simulink model "ejh42"  (Simulink 3.00)
settings: Solver=ode45  StartTime=0.0  StopTime=10.0  RelTol=1e-3
settings Model: LastModifiedBy=Administrador

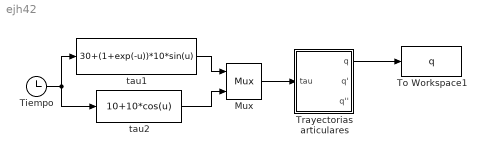
== system ejh42 ==
  Mux : Mux  Inputs=2
      settings: DisplayOption=none
  Tiempo : Clock
      settings: DisplayTime=off  Decimation=10
  To Workspace1 : ToWorkspace  VariableName=q  SampleTime=-1  SaveFormat=Matrix
  Trayectorias articulares : Subsystem  mask(Trayectorias articulares){dyn=[0 0 0 0 0 2 3 0 0 0 0 0 0 0 0 0 1 0 0 0; 0 3 0 0 0 1 1 0 0 0 0 0 0 0 0 0 1 0 0 0], grav=[0 -9.81 0], inivel=[0 0], inipos=[0 0]}
      mask prompts: dyn "Matriz de parámetros cinemáticos y dinámicos:"; grav "Vector aceleración de la gravedad:"; inivel "Velocidades articulares iniciales:"; inipos "Posiciones articulares iniciales:"
      mask help: Se calculan las trayectorias articulares (posiciones, velocidades y aceleraciones articulares) a partir de los pares aplicados al manipulador.
  tau1 : Fcn  Expr=30+(1+exp(-u))*10*sin(u)
  tau2 : Fcn  Expr=10+10*cos(u)
  wires:
  Mux/1 -> Trayectorias articulares/1(tau)
  Trayectorias articulares/1(q) -> To Workspace1/1
  Tiempo/1 -> tau1/1, tau2/1
  tau1/1 -> Mux/1
  tau2/1 -> Mux/2

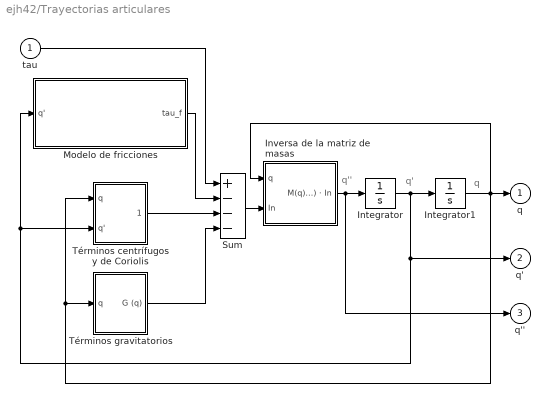
== system ejh42/Trayectorias articulares ==
  note: q
  note: q''
  note: q'
  tau : Inport  Port=1  PortWidth=-1  SampleTime=-1  DataType=auto
      settings: SignalType=auto
  Integrator : Integrator  ExternalReset=none  InitialConditionSource=internal  InitialCondition=inivel(:)  LimitOutput=off  UpperSaturationLimit=inf  LowerSaturationLimit=-inf  ShowSaturationPort=off  ShowStatePort=off  AbsoluteTolerance=auto
  Integrator1 : Integrator  ExternalReset=none  InitialConditionSource=internal  InitialCondition=inipos(:)  LimitOutput=off  UpperSaturationLimit=inf  LowerSaturationLimit=-inf  ShowSaturationPort=off  ShowStatePort=off  AbsoluteTolerance=auto
  Inversa de la matriz de masas : Subsystem  mask(Término de Coriolis){dyn=dyn}
      mask prompts: dyn "Matriz de parámetros dinámicos:"
      mask help: Este bloque devuelve el par correspondiente al término de Coriolis.
      mask Help: A este bloque hay que darle tres parámetros: 1) La matriz de parámetros dinámicos del manipulador de acuerdo con el formato que se explica en la sección "dyn" del Apéndice, 2) Un vector columna correspondiente a la aceleración de la gravedad, y 3) Un vector columna correspondiente a las fuerzas externas.
  Modelo de fricciones : Subsystem  mask(Modelo de fricciones (viscosa y de Coriolis)){G=dyn (:,17), b=dyn (:,18), tcp=dyn (:,19), tcm=dyn (:,20)}
      mask prompts: G "Factores de reducción (G):"; b "Fricciones viscosas, referidas al motor:"; tcp "Fricciones de Coulomb (rotación +), referidas al motor:"; tcm "Fricciones de Coulomb (rotación -), referidas al motor:"
      mask help:
      | Este bloque calcula el par correspondiente a la fricciones viscosa y de Coulomb. Para ello se emplea un determinado modelo para dichas fricciones:
      |            B·q' + Tc + ,  si q'>0
      |            B·q' + Tc - ,  si q'<0
      mask Display:
      | disp('B·q'' + Tc + ,  si q''>0\n')
      | disp('\nB·q'' + Tc - ,  si q''<0')
  Sum : Sum  Inputs=+---  SaturateOnIntegerOverflow=on
  Términos gravitatorios : Subsystem  mask(Término de Coriolis){dyn=dyn, grav=grav}
      mask prompts: dyn "Matriz de parámetros dinámicos:"; grav "Vector aceleración de la gravedad:"
      mask help: Este bloque devuelve el par correspondiente al término de Coriolis.
      mask Help: A este bloque hay que darle tres parámetros: 1) La matriz de parámetros dinámicos del manipulador de acuerdo con el formato que se explica en la sección "dyn" del Apéndice, 2) Un vector columna correspondiente a la aceleración de la gravedad, y 3) Un vector columna correspondiente a las fuerzas externas.
  Términos centrífugos y de Coriolis : Subsystem  mask(Término de Coriolis){dyn=dyn}
      mask prompts: dyn "Matriz de parámetros dinámicos:"
      mask help: Este bloque devuelve el par correspondiente al término de Coriolis.
      mask Help: A este bloque hay que darle tres parámetros: 1) La matriz de parámetros dinámicos del manipulador de acuerdo con el formato que se explica en la sección "dyn" del Apéndice, 2) Un vector columna correspondiente a la aceleración de la gravedad, y 3) Un vector columna correspondiente a las fuerzas externas.
  q : Outport  Port=1  InitialOutput=0
  q' : Outport  Port=2  InitialOutput=0
  q'' : Outport  Port=3  InitialOutput=0
  wires:
  Integrator1/1 -> q/1, Inversa de la matriz de masas/1(q), Términos centrífugos y de Coriolis/1(q), Términos gravitatorios/1(q)
  Integrator/1 -> Integrator1/1, q'/1, Términos centrífugos y de Coriolis/2(q'), Modelo de fricciones/1(q')
  Sum/1 -> Inversa de la matriz de masas/2(In)
  tau/1 -> Sum/1
  Inversa de la matriz de masas/1(M(q)^(-1) · In) -> Integrator/1, q''/1
  Términos gravitatorios/1(G (q)) -> Sum/4
  Términos centrífugos y de Coriolis/1(V (q,q')) -> Sum/3
  Modelo de fricciones/1(tau_f) -> Sum/2

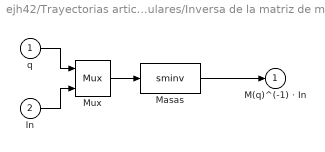
== system ejh42/Trayectorias articulares/Inversa de la matriz de masas ==
  q : Inport  Port=1  PortWidth=-1  SampleTime=-1  DataType=auto
      settings: SignalType=auto
  In : Inport  Port=2  PortWidth=-1  SampleTime=-1  DataType=auto
      settings: SignalType=auto
  Masas : S-Function  FunctionName=sminv  Parameters=dyn  PortCounts=[]  SFunctionModules=''
  Mux : Mux  Inputs=2
      settings: DisplayOption=none
  M(q)^(-1) · In : Outport  Port=1  InitialOutput=0
  wires:
  Mux/1 -> Masas/1
  q/1 -> Mux/1
  In/1 -> Mux/2
  Masas/1 -> M(q)^(-1) · In/1

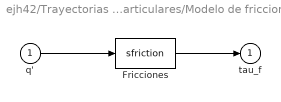
== system ejh42/Trayectorias articulares/Modelo de fricciones ==
  q' : Inport  Port=1  PortWidth=-1  SampleTime=-1  DataType=auto
      settings: SignalType=auto
  Fricciones : S-Function  FunctionName=sfriction  Parameters=G,b,tcp,tcm  PortCounts=[]  SFunctionModules=''
  tau_f : Outport  Port=1  InitialOutput=0
  wires:
  q'/1 -> Fricciones/1
  Fricciones/1 -> tau_f/1

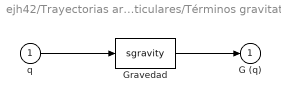
== system ejh42/Trayectorias articulares/Términos gravitatorios ==
  q : Inport  Port=1  PortWidth=-1  SampleTime=-1  DataType=auto
      settings: SignalType=auto
  Gravedad : S-Function  FunctionName=sgravity  Parameters=dyn,grav  PortCounts=[]  SFunctionModules=''
  G (q) : Outport  Port=1  InitialOutput=0
  wires:
  q/1 -> Gravedad/1
  Gravedad/1 -> G (q)/1

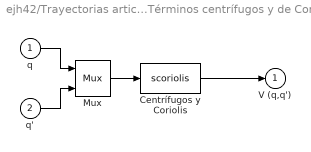
== system ejh42/Trayectorias articulares/Términos centrífugos y de Coriolis ==
  q : Inport  Port=1  PortWidth=-1  SampleTime=-1  DataType=auto
      settings: SignalType=auto
  q' : Inport  Port=2  PortWidth=-1  SampleTime=-1  DataType=auto
      settings: SignalType=auto
  Centrífugos y Coriolis : S-Function  FunctionName=scoriolis  Parameters=dyn  PortCounts=[]  SFunctionModules=''
  Mux : Mux  Inputs=2
      settings: DisplayOption=none
  V (q,q') : Outport  Port=1  InitialOutput=0
  wires:
  Mux/1 -> Centrífugos y Coriolis/1
  q/1 -> Mux/1
  q'/1 -> Mux/2
  Centrífugos y Coriolis/1 -> V (q,q')/1
